simulink model "altitude_smoothening_Harness1"  (R2025b)
settings: Solver=FixedStepDiscrete  StartTime=0.0  StopTime=10.0  FixedStep=0.1  RelTol=1e-3
settings OptimizationCC: DefaultParameterBehavior=Inlined  EnhancedBackFolding=on  PassReuseOutputArgsAs=Individual arguments  ZeroExternalMemoryAtStartup=off  ZeroInternalMemoryAtStartup=off  OptimizeBlockOrder=speed  DifferentSizesBufferReuse=on  OptimizationCustomize=off  EfficientTunableParamExpr=on
settings DebuggingCC: ParameterTunabilityLossMsg=error
settings SFSimCC: MATLABDynamicMemAlloc=off
settings RTWCC: SystemTargetFile=ert.tlc  GenCodeOnly=on  TemplateMakefile=ert_default_tmf  Description=Embedded Coder
settings CodeAppCC: ForceParamTrailComments=on  IgnoreCustomStorageClasses=off  MaxIdLength=128.0  OperatorAnnotations=on  SimulinkDataObjDesc=on  SFDataObjDesc=on  InsertBlockDesc=on  InternalIdentifier=Classic
settings ERTTargetCC: ERTCustomFileTemplate=example_file_process.tlc  TargetLangStandard=C99 (ISO)  GenerateSampleERTMain=on

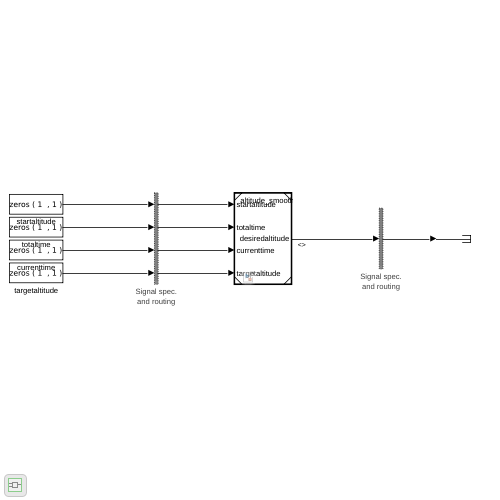
[thumbnail: Simulink's stored preview of the top-level diagram]
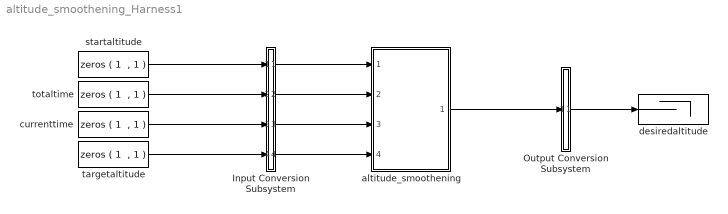
== system altitude_smoothening_Harness1 ==
  Input Conversion Subsystem : Subsystem  Tag=__SLT_ICS__  Description=|
      | Signal spec.
      | and routing
      settings: AttributesFormatString=%<Description>
  Output Conversion Subsystem : Subsystem  Tag=__SLT_OCS__  Description=|
      | Signal spec.
      | and routing
      settings: AttributesFormatString=%<Description>
  altitude_smoothening : ModelReference  ModelNameDialog=altitude_smoothening  SimulationMode=Normal  ModelReferenceVersion=1.33
  currenttime : Constant  Value="zeros ( 1  , 1 )"  OutDataTypeStr=uint8  SampleTime=0.1
  desiredaltitude : Terminator
  startaltitude : Constant  Value="zeros ( 1  , 1 )"  OutDataTypeStr=uint8  SampleTime=0.1
  targetaltitude : Constant  Value="zeros ( 1  , 1 )"  OutDataTypeStr=uint8  SampleTime=0.1
  totaltime : Constant  Value="zeros ( 1  , 1 )"  OutDataTypeStr=uint8  SampleTime=0.1
  wires:
  startaltitude/1 -> Input Conversion Subsystem/1(Inport_1)
  totaltime/1 -> Input Conversion Subsystem/2(Inport_2)
  currenttime/1 -> Input Conversion Subsystem/3(Inport_3)
  targetaltitude/1 -> Input Conversion Subsystem/4(Inport_4)
  Output Conversion Subsystem/1(Outport_1) -> desiredaltitude/1
  Input Conversion Subsystem/1(Outport_1) -> altitude_smoothening/1
  Input Conversion Subsystem/2(Outport_2) -> altitude_smoothening/2
  Input Conversion Subsystem/3(Outport_3) -> altitude_smoothening/3
  Input Conversion Subsystem/4(Outport_4) -> altitude_smoothening/4
  altitude_smoothening/1 -> Output Conversion Subsystem/1(Inport_1)

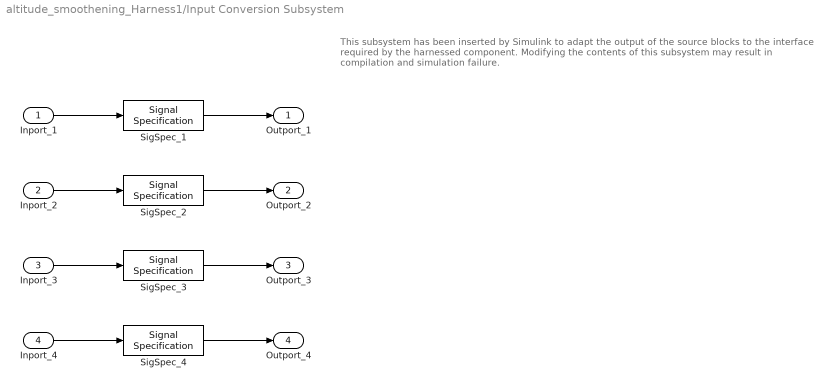
== system altitude_smoothening_Harness1/Input Conversion Subsystem ==
  note: This subsystem has been inserted by Simulink to adapt the output of the source blocks to the interface required by the harnessed component.
      |  Modifying the contents of this subsystem may result in compilation and simulation failure.
  Inport_1 : Inport
  Inport_2 : Inport  Port=2
  Inport_3 : Inport  Port=3
  Inport_4 : Inport  Port=4
  SigSpec_{1..4} (4 alike) : SignalSpecification  OutDataTypeStr=uint8  Dimensions=[1]  SampleTime=0.1
  Outport_1 : Outport
  Outport_2 : Outport  Port=2
  Outport_3 : Outport  Port=3
  Outport_4 : Outport  Port=4
  wires:
  SigSpec_1/1 -> Outport_1/1
  Inport_1/1 -> SigSpec_1/1
  SigSpec_2/1 -> Outport_2/1
  Inport_2/1 -> SigSpec_2/1
  SigSpec_3/1 -> Outport_3/1
  Inport_3/1 -> SigSpec_3/1
  SigSpec_4/1 -> Outport_4/1
  Inport_4/1 -> SigSpec_4/1

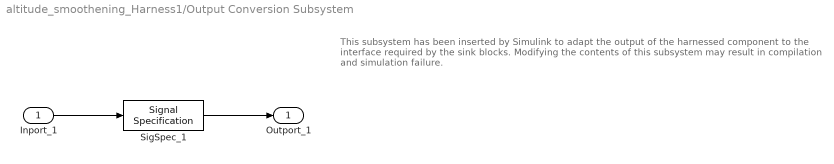
== system altitude_smoothening_Harness1/Output Conversion Subsystem ==
  note: This subsystem has been inserted by Simulink to adapt the output of the harnessed component to the interface required by the sink blocks.
      |  Modifying the contents of this subsystem may result in compilation and simulation failure.
  Inport_1 : Inport
  SigSpec_1 : SignalSpecification  OutDataTypeStr=uint16  Dimensions=[1]  SampleTime=0.1
  Outport_1 : Outport
  wires:
  Inport_1/1 -> SigSpec_1/1
  SigSpec_1/1 -> Outport_1/1
